simulink model "test_7x7x7_timing"  (R2013b)
settings: Solver=ode3  SolverMode=SingleTasking  StartTime=0.0  StopTime=inf  RelTol=1e-3
InitFcn:
  | close all
model workspace (MAT data in the model file):
  dt = 0.003
libraries: arduinolib x97, simulink x8, rtwinlib x1
settings Model: ExtModeTrigDuration=2  Creator=sbiagion  LastModifiedBy=sbiagion
settings DataIOCC: SignalLoggingSaveFormat=ModelDataLogs
settings OptimizationCC: OptimizeModelRefInitCode=on  LifeSpan=1
settings DebuggingCC: SolverPrmCheckMsg=none  MultiTaskDSMMsg=warning  MultiTaskCondExecSysMsg=none
settings HardwareCC: ProdBitPerInt=16  ProdBitPerPointer=8  ProdIntDivRoundTo=Zero  ProdEndianess=LittleEndian  ProdWordSize=8  ProdHWDeviceType=Atmel->AVR
settings RTWCC: SystemTargetFile=realtime.tlc  GenerateMakefile=off  TemplateMakefile=realtime.tmf  Description=Run on Target Hardware  RTWVerbose=off  ProcessScript=realtime_make_rtw_hook  IncludeERTFirstTime=on
settings STFCustomTargetCC: TargetLibSuffix=.a  GenerateSampleERTMain=on  ERTCustomFileBanners=on  SupportNonInlinedSFcns=off  SupportVariableSizeSignals=on  MATLABClassNameForMDSCustomization=Simulink.SoftwareTarget.ERTCustomization  GRTInterface=off  SystemTargetFile=realtime.tlc
settings ERTTargetCC: CodeReplacementLibrary=ANSI_C  GenerateSampleERTMain=on  ParMdlRefBuildCompliant=off  CompOptLevelCompliant=off  ConcurrentExecutionCompliant=off  CombineOutputUpdateFcns=off  ERTFirstTimeCompliant=off  SupportContinuousTime=on  SupportVariableSizeSignals=on  ModelStepFunctionPrototypeControlCompliant=off  CPPClassGenCompliant=off  ExtMode=on  ExtModeTransport=3  ExtModeMexFile=ext_serial_win32_comm  ExtModeMexArgs=0 18 115200  InlinedParameterPlacement=NonHierarchical  ERTSrcFileBannerTemplate=realtime_code_template.cgt  ERTHdrFileBannerTemplate=realtime_code_template.cgt  ERTDataSrcFileTemplate=realtime_code_template.cgt  ERTDataHdrFileTemplate=realtime_code_template.cgt  ERTCustomFileTemplate=realtime_file_process.tlc

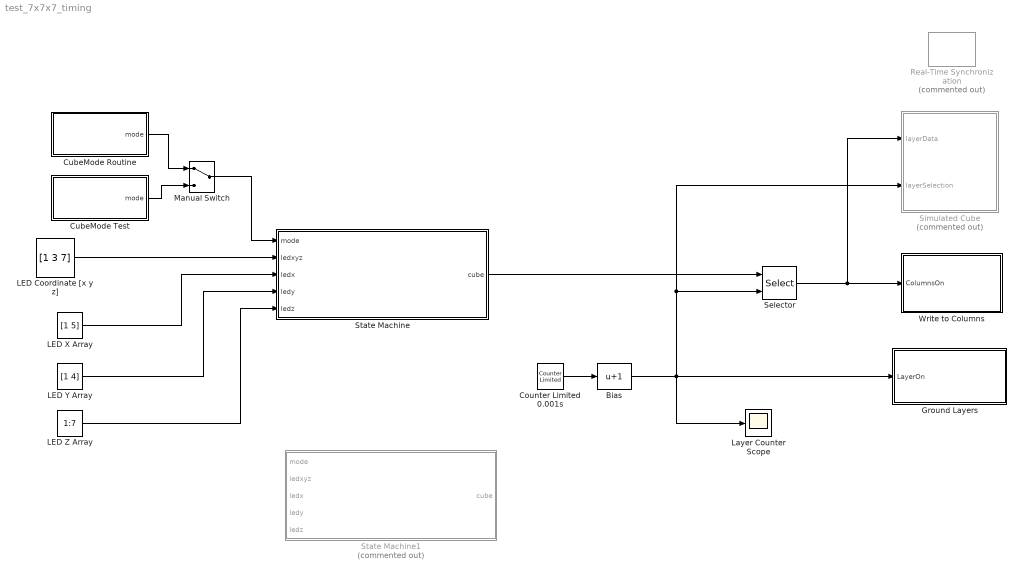
== system test_7x7x7_timing ==
  Bias : Bias  Bias=1
  Counter Limited 0.001s : simulink/Sources/Counter Limited  uplimit=6  tsamp=dt
  CubeMode Routine : Stateflow chart  TreatAsAtomicUnit=on
  CubeMode Test : Stateflow chart  TreatAsAtomicUnit=on
  Ground Layers : Subsystem
  LED Coordinate [x y z] : Constant  Value=[1 3 7]  SampleTime=-1
  LED X Array : Constant  Value=[1 5]
  LED Y Array : Constant  Value=[1 4]
  LED Z Array : Constant  Value=1:7
  Layer Counter Scope : Scope
      settings: TimeRange=20  YMin=-1  YMax=7
  Manual Switch : ManualSwitch
  Real-Time Synchronization : rtwinlib/Real-Time Synchronization  Commented=on  SampleTime=1  MaxMissedTicks=1000  ShowMissedTicks=off  YieldWhenWaiting=on
  Selector : Selector  NumberOfDimensions=3  InputPortWidth=3  SampleTime=dt  IndexOptions=Select all,Select all,Index vector (port)  Indices=1:7,1:7,1  OutputSizes=1,1,1
  Simulated Cube : MATLAB Function  Commented=on  TreatAsAtomicUnit=on
  State Machine : Stateflow chart  TreatAsAtomicUnit=on  SystemSampleTime=0.1
  State Machine1 : Stateflow chart  Commented=on  TreatAsAtomicUnit=on  SystemSampleTime=0.1
  Write to Columns : Subsystem
  wires:
  CubeMode Test/1(mode) -> Manual Switch/2
  State Machine/1(cube) -> Selector/1
  Counter Limited 0.001s/1 -> Bias/1
  LED Coordinate [x y z]/1 -> State Machine/2(ledxyz)
  Selector/1 -> Simulated Cube/1(layerData), Write to Columns/1(ColumnsOn)
  LED X Array/1 -> State Machine/3(ledx)
  LED Y Array/1 -> State Machine/4(ledy)
  LED Z Array/1 -> State Machine/5(ledz)
  Bias/1 -> Simulated Cube/2(layerSelection), Selector/2, Ground Layers/1(LayerOn), Layer Counter Scope/1
  CubeMode Routine/1(mode) -> Manual Switch/1
  Manual Switch/1 -> State Machine/1(mode)

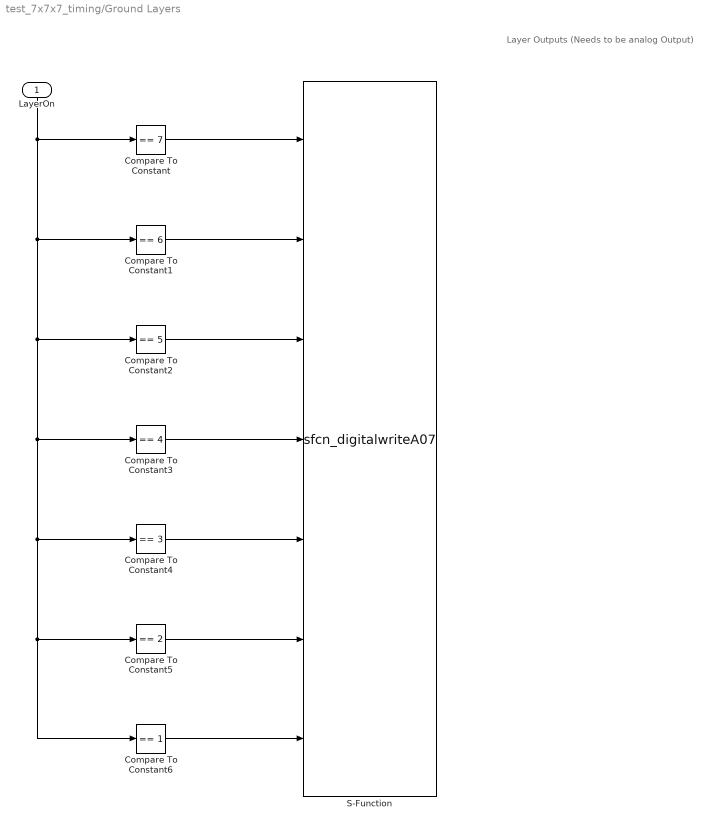
== system test_7x7x7_timing/Ground Layers ==
  note: Layer Outputs (Needs to be analog Output)
  LayerOn : Inport
  Compare To Constant : simulink/Logic and Bit Operations/Compare To Constant  relop===  const=7  OutDataTypeStr=uint8
  Compare To Constant1 : simulink/Logic and Bit Operations/Compare To Constant  relop===  const=6  OutDataTypeStr=uint8
  Compare To Constant2 : simulink/Logic and Bit Operations/Compare To Constant  relop===  const=5  OutDataTypeStr=uint8
  Compare To Constant3 : simulink/Logic and Bit Operations/Compare To Constant  relop===  const=4  OutDataTypeStr=uint8
  Compare To Constant4 : simulink/Logic and Bit Operations/Compare To Constant  relop===  const=3  OutDataTypeStr=uint8
  Compare To Constant5 : simulink/Logic and Bit Operations/Compare To Constant  relop===  const=2  OutDataTypeStr=uint8
  Compare To Constant6 : simulink/Logic and Bit Operations/Compare To Constant  relop===  const=1  OutDataTypeStr=uint8
  S-Function : S-Function  FunctionName=sfcn_digitalwriteA07  Parameters=0  EnableBusSupport=off
  wires:
  LayerOn/1 -> Compare To Constant6/1, Compare To Constant5/1, Compare To Constant4/1, Compare To Constant3/1, Compare To Constant2/1, Compare To Constant1/1, Compare To Constant/1
  Compare To Constant/1 -> S-Function/1
  Compare To Constant1/1 -> S-Function/2
  Compare To Constant2/1 -> S-Function/3
  Compare To Constant3/1 -> S-Function/4
  Compare To Constant4/1 -> S-Function/5
  Compare To Constant5/1 -> S-Function/6
  Compare To Constant6/1 -> S-Function/7

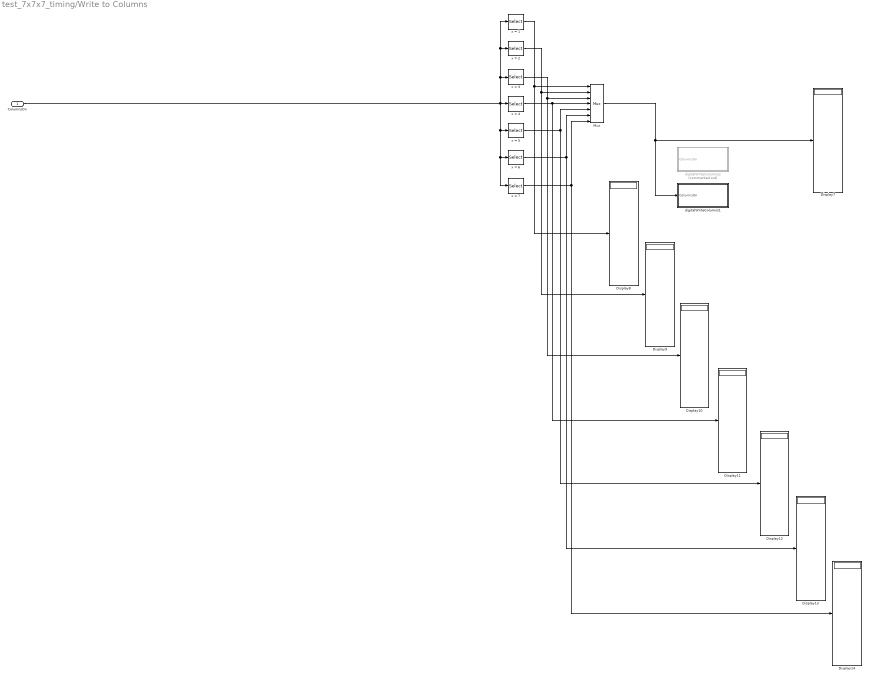
== system test_7x7x7_timing/Write to Columns ==
  ColumnsOn : Inport
  Display{7..14} (8 alike) : Display
  Mux : Mux  Inputs=7
  digitalWriteColumns1 : Subsystem
  digitalWriteColumns2 : Subsystem  Commented=on
  x = 1 : Selector  NumberOfDimensions=2  InputPortWidth=49  IndexOptions=Index vector (dialog),Select all  Indices=1,1  OutputSizes=1,1
  x = 2 : Selector  NumberOfDimensions=2  InputPortWidth=49  IndexOptions=Index vector (dialog),Select all  Indices=2,2  OutputSizes=1,1
  x = 3 : Selector  NumberOfDimensions=2  InputPortWidth=49  IndexOptions=Index vector (dialog),Select all  Indices=3,3  OutputSizes=1,1
  x = 4 : Selector  NumberOfDimensions=2  InputPortWidth=49  IndexOptions=Index vector (dialog),Select all  Indices=4,4  OutputSizes=1,1
  x = 5 : Selector  NumberOfDimensions=2  InputPortWidth=49  IndexOptions=Index vector (dialog),Select all  Indices=5,5  OutputSizes=1,1
  x = 6 : Selector  NumberOfDimensions=2  InputPortWidth=49  IndexOptions=Index vector (dialog),Select all  Indices=6,6  OutputSizes=1,1
  x = 7 : Selector  NumberOfDimensions=2  InputPortWidth=49  IndexOptions=Index vector (dialog),Select all  Indices=7,7  OutputSizes=1,1
  wires:
  x = 1/1 -> Display8/1, Mux/1
  x = 2/1 -> Display9/1, Mux/2
  x = 3/1 -> Mux/3, Display10/1
  ColumnsOn/1 -> x = 1/1, x = 2/1, x = 3/1, x = 4/1, x = 5/1, x = 7/1, x = 6/1
  x = 6/1 -> Mux/6, Display13/1
  x = 5/1 -> Mux/5, Display12/1
  Mux/1 -> digitalWriteColumns1/1(ColumnsOn), Display7/1
  x = 7/1 -> Mux/7, Display14/1
  x = 4/1 -> Mux/4, Display11/1

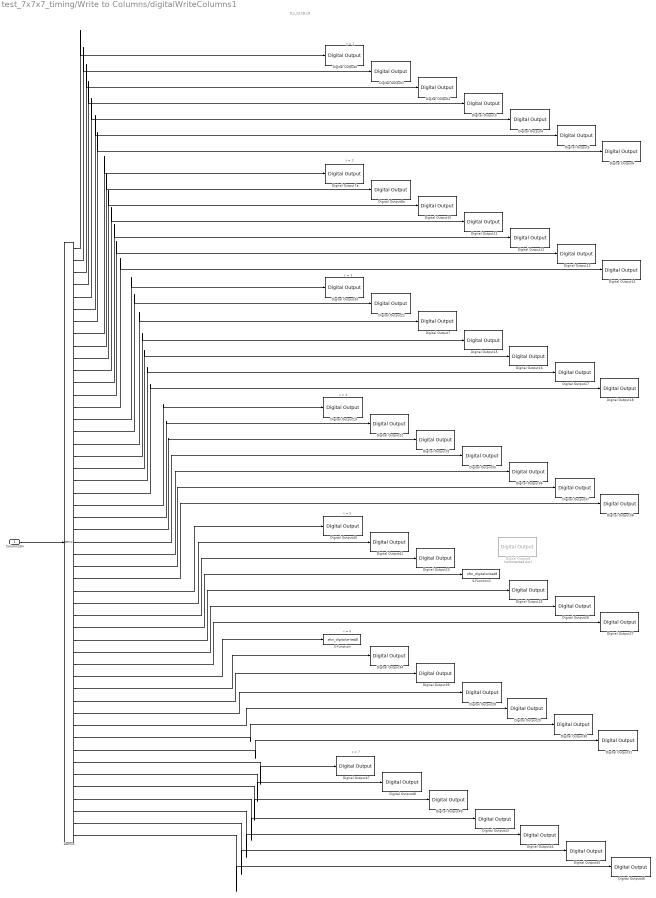
== system test_7x7x7_timing/Write to Columns/digitalWriteColumns1 ==
  note: 0,1,13,18,19
  note: x = 7
  note: x = 6
  note: x = 5
  note: x = 4
  note: x = 3
  note: x = 2
  note: x = 1
  ColumnsOn : Inport
  Demux : Demux  Outputs=49
  Digital Output0 : arduinolib/Digital Output  pinNumber=38
  Digital Output1 : arduinolib/Digital Output  pinNumber=40
  Digital Output10 : arduinolib/Digital Output  pinNumber=44
  Digital Output11 : arduinolib/Digital Output  pinNumber=35
  Digital Output12 : arduinolib/Digital Output  pinNumber=45
  Digital Output13 : arduinolib/Digital Output  pinNumber=32
  Digital Output14 : arduinolib/Digital Output  pinNumber=46
  Digital Output15 : arduinolib/Digital Output  pinNumber=48
  Digital Output16 : arduinolib/Digital Output  pinNumber=31
  Digital Output17 : arduinolib/Digital Output  pinNumber=49
  Digital Output18 : arduinolib/Digital Output  pinNumber=28
  Digital Output19 : arduinolib/Digital Output  pinNumber=50
  Digital Output2 : arduinolib/Digital Output  pinNumber=39
  Digital Output20 : arduinolib/Digital Output  pinNumber=33
  Digital Output21 : arduinolib/Digital Output  pinNumber=47
  Digital Output22 : arduinolib/Digital Output  pinNumber=29
  Digital Output23 : arduinolib/Digital Output  pinNumber=22
  Digital Output25 : arduinolib/Digital Output  pinNumber=25
  Digital Output26 : arduinolib/Digital Output  pinNumber=8
  Digital Output27 : arduinolib/Digital Output  pinNumber=24
  Digital Output28 : arduinolib/Digital Output  pinNumber=10
  Digital Output29 : arduinolib/Digital Output  pinNumber=4
  Digital Output3 : arduinolib/Digital Output  pinNumber=41
  Digital Output30 : arduinolib/Digital Output  pinNumber=9
  Digital Output31 : arduinolib/Digital Output  pinNumber=5
  Digital Output32 : arduinolib/Digital Output  pinNumber=51
  Digital Output34 : arduinolib/Digital Output  pinNumber=21
  Digital Output35 : arduinolib/Digital Output  pinNumber=26
  Digital Output36 : arduinolib/Digital Output  pinNumber=52
  Digital Output37 : arduinolib/Digital Output  pinNumber=27
  Digital Output38 : arduinolib/Digital Output  pinNumber=53
  Digital Output39 : arduinolib/Digital Output  pinNumber=3
  Digital Output4 : arduinolib/Digital Output  pinNumber=36
  Digital Output40 : arduinolib/Digital Output  pinNumber=23
  Digital Output41 : arduinolib/Digital Output  pinNumber=6
  Digital Output43 : arduinolib/Digital Output  pinNumber=11
  Digital Output44 : arduinolib/Digital Output  pinNumber=17
  Digital Output45 : arduinolib/Digital Output  pinNumber=12
  Digital Output46 : arduinolib/Digital Output  pinNumber=20
  Digital Output47 : arduinolib/Digital Output  pinNumber=15
  Digital Output48 : arduinolib/Digital Output  pinNumber=14
  Digital Output49 : arduinolib/Digital Output  pinNumber=16
  Digital Output5 : arduinolib/Digital Output  pinNumber=42
  Digital Output6 : arduinolib/Digital Output  pinNumber=37
  Digital Output7 : arduinolib/Digital Output  pinNumber=30
  Digital Output7a : arduinolib/Digital Output  pinNumber=43
  Digital Output8 : arduinolib/Digital Output  Commented=on  pinNumber=7
  Digital Output8a : arduinolib/Digital Output  pinNumber=34
  S-Function : S-Function  FunctionName=sfcn_digitalwriteA8  Parameters=0  EnableBusSupport=off
  S-Function1 : S-Function  FunctionName=sfcn_digitalwriteA9  Parameters=0  EnableBusSupport=off
  wires:
  Demux/4 -> Digital Output3/1
  ColumnsOn/1 -> Demux/1
  Demux/3 -> Digital Output2/1
  Demux/2 -> Digital Output1/1
  Demux/1 -> Digital Output0/1
  Demux/7 -> Digital Output6/1
  Demux/6 -> Digital Output5/1
  Demux/5 -> Digital Output4/1
  Demux/11 -> Digital Output11/1
  Demux/10 -> Digital Output10/1
  Demux/9 -> Digital Output8a/1
  Demux/8 -> Digital Output7a/1
  Demux/14 -> Digital Output14/1
  Demux/13 -> Digital Output13/1
  Demux/12 -> Digital Output12/1
  Demux/18 -> Digital Output15/1
  Demux/17 -> Digital Output7/1
  Demux/16 -> Digital Output21/1
  Demux/15 -> Digital Output20/1
  Demux/21 -> Digital Output18/1
  Demux/20 -> Digital Output17/1
  Demux/19 -> Digital Output16/1
  Demux/25 -> Digital Output35/1
  Demux/24 -> Digital Output32/1
  Demux/23 -> Digital Output22/1
  Demux/22 -> Digital Output19/1
  Demux/28 -> Digital Output38/1
  Demux/27 -> Digital Output37/1
  Demux/26 -> Digital Output36/1
  Demux/32 -> S-Function1/1
  Demux/31 -> Digital Output23/1
  Demux/30 -> Digital Output41/1
  Demux/29 -> Digital Output40/1
  Demux/35 -> Digital Output27/1
  Demux/34 -> Digital Output26/1
  Demux/33 -> Digital Output25/1
  Demux/39 -> Digital Output28/1
  Demux/38 -> Digital Output39/1
  Demux/37 -> Digital Output34/1
  Demux/36 -> S-Function/1
  Demux/42 -> Digital Output31/1
  Demux/41 -> Digital Output30/1
  Demux/40 -> Digital Output29/1
  Demux/46 -> Digital Output43/1
  Demux/45 -> Digital Output49/1
  Demux/44 -> Digital Output48/1
  Demux/43 -> Digital Output47/1
  Demux/49 -> Digital Output46/1
  Demux/48 -> Digital Output45/1
  Demux/47 -> Digital Output44/1

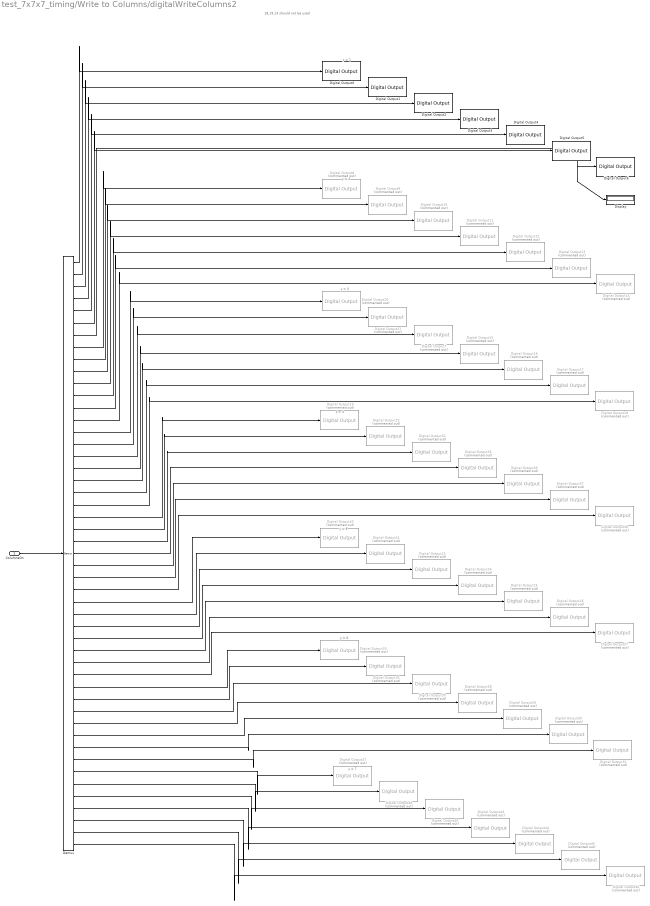
== system test_7x7x7_timing/Write to Columns/digitalWriteColumns2 ==
  note: y = 1
  note: y = 2
  note: y = 3
  note: y = 4
  note: y = 5
  note: y = 6
  note: y = 7
  note: 18,19,13 should not be used
  ColumnsOn : Inport
  Demux : Demux  Outputs=49
  Digital Output0 : arduinolib/Digital Output  pinNumber=2
  Digital Output1 : arduinolib/Digital Output  pinNumber=3
  Digital Output10 : arduinolib/Digital Output  Commented=on  pinNumber=9
  Digital Output11 : arduinolib/Digital Output  Commented=on  pinNumber=10
  Digital Output12 : arduinolib/Digital Output  Commented=on  pinNumber=11
  Digital Output13 : arduinolib/Digital Output  Commented=on  pinNumber=49
  Digital Output14 : arduinolib/Digital Output  Commented=on  pinNumber=50
  Digital Output15 : arduinolib/Digital Output  Commented=on  pinNumber=15
  Digital Output16 : arduinolib/Digital Output  Commented=on  pinNumber=16
  Digital Output17 : arduinolib/Digital Output  Commented=on  pinNumber=17
  Digital Output18 : arduinolib/Digital Output  Commented=on  pinNumber=18
  Digital Output19 : arduinolib/Digital Output  Commented=on  pinNumber=19
  Digital Output2 : arduinolib/Digital Output  pinNumber=4
  Digital Output20 : arduinolib/Digital Output  Commented=on  pinNumber=12
  Digital Output21 : arduinolib/Digital Output  Commented=on  pinNumber=51
  Digital Output22 : arduinolib/Digital Output  Commented=on  pinNumber=20
  Digital Output23 : arduinolib/Digital Output  Commented=on  pinNumber=28
  Digital Output24 : arduinolib/Digital Output  Commented=on  pinNumber=29
  Digital Output25 : arduinolib/Digital Output  Commented=on  pinNumber=30
  Digital Output26 : arduinolib/Digital Output  Commented=on  pinNumber=31
  Digital Output27 : arduinolib/Digital Output  Commented=on  pinNumber=32
  Digital Output28 : arduinolib/Digital Output  Commented=on  pinNumber=36
  Digital Output29 : arduinolib/Digital Output  Commented=on  pinNumber=37
  Digital Output3 : arduinolib/Digital Output  pinNumber=5
  Digital Output30 : arduinolib/Digital Output  Commented=on  pinNumber=38
  Digital Output31 : arduinolib/Digital Output  Commented=on  pinNumber=39
  Digital Output32 : arduinolib/Digital Output  Commented=on  pinNumber=21
  Digital Output33 : arduinolib/Digital Output  Commented=on  pinNumber=33
  Digital Output34 : arduinolib/Digital Output  Commented=on  pinNumber=34
  Digital Output35 : arduinolib/Digital Output  Commented=on  pinNumber=22
  Digital Output36 : arduinolib/Digital Output  Commented=on  pinNumber=23
  Digital Output37 : arduinolib/Digital Output  Commented=on  pinNumber=24
  Digital Output38 : arduinolib/Digital Output  Commented=on  pinNumber=25
  Digital Output39 : arduinolib/Digital Output  Commented=on  pinNumber=35
  Digital Output4 : arduinolib/Digital Output  pinNumber=6
  Digital Output40 : arduinolib/Digital Output  Commented=on  pinNumber=26
  Digital Output41 : arduinolib/Digital Output  Commented=on  pinNumber=27
  Digital Output43 : arduinolib/Digital Output  Commented=on  pinNumber=43
  Digital Output44 : arduinolib/Digital Output  Commented=on  pinNumber=44
  Digital Output45 : arduinolib/Digital Output  Commented=on  pinNumber=45
  Digital Output46 : arduinolib/Digital Output  Commented=on  pinNumber=46
  Digital Output47 : arduinolib/Digital Output  Commented=on  pinNumber=40
  Digital Output48 : arduinolib/Digital Output  Commented=on  pinNumber=41
  Digital Output49 : arduinolib/Digital Output  Commented=on  pinNumber=42
  Digital Output5 : arduinolib/Digital Output  pinNumber=7
  Digital Output6 : arduinolib/Digital Output  pinNumber=53
  Digital Output7 : arduinolib/Digital Output  Commented=on  pinNumber=14
  Digital Output8 : arduinolib/Digital Output  Commented=on  pinNumber=7
  Digital Output9 : arduinolib/Digital Output  Commented=on  pinNumber=8
  Display : Display
  wires:
  Demux/47 -> Digital Output44/1
  Demux/48 -> Digital Output45/1
  Demux/49 -> Digital Output46/1
  Demux/43 -> Digital Output47/1
  Demux/44 -> Digital Output48/1
  Demux/45 -> Digital Output49/1
  Demux/46 -> Digital Output43/1
  Demux/40 -> Digital Output29/1
  Demux/41 -> Digital Output30/1
  Demux/42 -> Digital Output31/1
  Demux/36 -> Digital Output33/1
  Demux/37 -> Digital Output34/1
  Demux/38 -> Digital Output39/1
  Demux/39 -> Digital Output28/1
  Demux/33 -> Digital Output25/1
  Demux/34 -> Digital Output26/1
  Demux/35 -> Digital Output27/1
  Demux/29 -> Digital Output40/1
  Demux/30 -> Digital Output41/1
  Demux/31 -> Digital Output23/1
  Demux/32 -> Digital Output24/1
  Demux/26 -> Digital Output36/1
  Demux/27 -> Digital Output37/1
  Demux/28 -> Digital Output38/1
  Demux/22 -> Digital Output19/1
  Demux/23 -> Digital Output22/1
  Demux/24 -> Digital Output32/1
  Demux/25 -> Digital Output35/1
  Demux/19 -> Digital Output16/1
  Demux/20 -> Digital Output17/1
  Demux/21 -> Digital Output18/1
  Demux/15 -> Digital Output20/1
  Demux/16 -> Digital Output21/1
  Demux/17 -> Digital Output7/1
  Demux/18 -> Digital Output15/1
  Demux/12 -> Digital Output12/1
  Demux/13 -> Digital Output13/1
  Demux/14 -> Digital Output14/1
  Demux/8 -> Digital Output8/1
  Demux/9 -> Digital Output9/1
  Demux/10 -> Digital Output10/1
  Demux/11 -> Digital Output11/1
  Demux/5 -> Digital Output4/1
  Demux/6 -> Digital Output5/1
  Demux/7 -> Digital Output6/1, Display/1
  Demux/1 -> Digital Output0/1
  Demux/2 -> Digital Output1/1
  Demux/3 -> Digital Output2/1
  ColumnsOn/1 -> Demux/1
  Demux/4 -> Digital Output3/1

== stateflow chart test_7x7x7_timing/CubeMode Routine ==
  state InitializeOff
    entry:
    mode = 1;
  state StarMode
    % 0:30 End of Basic Stage and Start of Yoshi Ride
    entry:
    mode = 7;
  state HeartMode
    % 1:05 Start of Double Seesaw
    entry:
    mode = 8;
  state TurnOff
    % end at 2:05
    entry: mode = 1;
  state FireworksMode
    % 1:45 End of Seesaw, starting at 1:35
    entry:
    mode = 9;
  (default) -> InitializeOff : % turn on 30s before NXT moves
  InitializeOff -> StarMode : after(60,sec)
  StarMode -> HeartMode : after(35,sec)
  FireworksMode -> TurnOff : after(30,sec)
  HeartMode -> FireworksMode : after(30,sec)
  data: mode output

== matlab function test_7x7x7_timing/Simulated Cube ==
  data: layerData input; layerSelection input
function simulatedCube(layerData,layerSelection)

coder.extrinsic('set','drawnow');

persistent cube t;

if isempty(cube)
  nLEDpDim = 7;
  
  t = 0;
  cube.nLEDpDim = nLEDpDim;
  fh = figure;
  set(fh,'renderer','opengl'); % if you close the figure window while the
                               % simulation is running, MATLAB will crash.
  ah = axes;
  xlabel('x-axis');
  ylabel('y-axis');
  zlabel('z-axis');
  set(ah,...
    'xLim',[0 nLEDpDim+1],...
    'yLim',[0 nLEDpDim+1],...
    'zLim',[0 nLEDpDim+1]);
  view(3);
  axis vis3d;
  grid on;
  set(ah,'XTick',[0 1 2 3 4 5 6 7 8])
  set(ah,'YTick',[0 1 2 3 4 5 6 7 8])
  set(ah,'ZTick',[0 1 2 3 4 5 6 7 8])
  cube.LED = zeros(nLEDpDim,nLEDpDim,nLEDpDim);
  for i = 1:nLEDpDim^3
    cube.LED(i) = line(0,0,0,...
      'parent',ah,...
      'color',[0.8,0.1,0.1],...
      'visible','off',...
      'marker','.',...
      'markerSize',15);
  end
  for i = 1:nLEDpDim
    set(cube.LED(i,:,:),'xData',i);
    set(cube.LED(:,i,:),'yData',i);
    set(cube.LED(:,:,i),'zData',i);
  end
end

if ~mod(t,1)
  set(cube.LED(:,:,mod(int8(layerSelection)-1,cube.nLEDpDim)+1),...
    'visible','off');
  activeLayer = cube.LED(:,:,layerSelection);
  activeLED   = activeLayer(logical(layerData));
  set(activeLED,'visible','on');
  drawnow;
end
t = t + 1;

== stateflow chart test_7x7x7_timing/State Machine ==
  state AllOff
    % All LED's off
    entry: cube = false(7,7,7);
  state Star
    %Star
    state MoveAlongPlane
      state Normal2Y
        state MoveAlongY
          en:
          j = j+1;
          if j==8
          j = 1;
          end
        state DrawStarY
          entry:
          % draw star normal to Y-axis
          cube  = drawStar(2,j);
        (default) -> DrawStarY : {j = 1;}
        DrawStarY -> MoveAlongY : after(0.1,sec)
        MoveAlongY -> DrawStarY
      state Normal2X
        state MoveAlongX
          en:
          i = i+1;
          if i==8
          i = 1;
          end
        state DrawStarX
          entry:
          cube  = drawStar(1,i);
        (default) -> DrawStarX : {i = 1;}
        DrawStarX -> MoveAlongX : after(0.1,sec)
        MoveAlongX -> DrawStarX
      (default) -> Star.MoveAlongPlane.Normal2Y
      Star.MoveAlongPlane.Normal2Y -> Star.MoveAlongPlane.Normal2X : after(5,sec)
      Star.MoveAlongPlane.Normal2X -> Star.MoveAlongPlane.Normal2Y : after(5,sec)
    state RotateSprite
      state normalToY
        entry:
        cube = rotateSprite(cube,'z','y',rStep);
      state Wait1
      state normalToX
        entry:
        cube = rotateSprite(cube,'z','x',rStep);
      state Wait2
      (default) -> Wait1 : {% draw star normal to y-axis
          | cube  = drawStar(1,4);
          | rStep = 1;}
      Wait1 -> normalToY [order 1] : [after(0.7,sec)]
      normalToY -> Wait1 : {rStep = rStep + 1;}
      Wait1 -> (junction 429) [order 2] : [rStep == 9]
      (junction 430) -> Wait1 : {rStep = 1;}
      (junction 429) -> Wait2 : {rStep = 1;}
      Wait2 -> (junction 430) [order 1] : [rStep == 9]
      Wait2 -> normalToX [order 2] : [after(0.7,sec)]
      normalToX -> Wait2 : {rStep = rStep + 1}
    (default) -> MoveAlongPlane
    MoveAlongPlane -> RotateSprite : after(20,sec)
  state Heart
    %Star
    state Normal2Y
      state drawNormal2Y
        entry: cube = drawHeart(2,4);
      state heartBeat
        entry: cube = drawHeartBeat(2,4);
      (default) -> drawNormal2Y
      drawNormal2Y -> Heart.Normal2Y.heartBeat : after(1.5,sec)
      Heart.Normal2Y.heartBeat -> drawNormal2Y : after(0.5,sec)
    state Normal2X
      state drawNormal2X
        entry: cube = drawHeart(1,4);
      state heartBeat
        entry: cube = drawHeartBeat(1,4);
      (default) -> drawNormal2X
      drawNormal2X -> Heart.Normal2X.heartBeat : after(1.5,sec)
      Heart.Normal2X.heartBeat -> drawNormal2X : after(0.5,sec)
    (default) -> Heart.Normal2Y
    Heart.Normal2Y -> Heart.Normal2X : after(10,sec)
    Heart.Normal2X -> Heart.Normal2Y : after(10,sec)
  state Firecrackers
    state LongWait
    state EvolveAnimation
      entry:
      cube = fireworks(cube,rStep,exp);
      exit:
      rStep = mod(rStep,21)+1;
    state ShortWait
      % Explosion
    (default) -> LongWait : {cube  = false(7,7,7);
        | exp = drawExplosion;
        | rStep = 1;}
    EvolveAnimation -> ShortWait [order 2] : [rStep > 8 && rStep < 15]
    LongWait -> EvolveAnimation : [after(0.1,sec)]
    ShortWait -> EvolveAnimation : [after(0.10,sec)]
    EvolveAnimation -> LongWait [order 1] : [rStep < 9 || rStep >14]
  state debug
  (default) -> (junction 73) : {cube = false(7,7,7);}
  (junction 69) -> (junction 73)
  (junction 73) -> (junction 402)
  (junction 400) -> (junction 69)
  (junction 402) -> AllOff [order 1] : [mode==1]
  (junction 402) -> (junction 455) [order 2]
  AllOff -> (junction 400) : [mode~=1]
  (junction 404) -> (junction 400)
  (junction 455) -> Star [order 1] : [mode==7]
  Star -> (junction 404) : [mode~=7]
  (junction 455) -> (junction 586) [order 2]
  (junction 585) -> (junction 404)
  (junction 586) -> Heart [order 1] : [mode==8]
  Heart -> (junction 585) : [mode~=8]
  (junction 586) -> (junction 470) [order 2]
  (junction 464) -> (junction 585)
  (junction 470) -> Firecrackers [order 1] : [mode==9]
  Firecrackers -> (junction 464) : [mode~=9]
  (junction 470) -> debug [order 2]
  data: cubeout function_output; axis function_input; coord function_input; bin function_input; rotationAxis function_input; normalAxis function_input; step function_input; b function_output; cubeout function_output; axis function_input; coord function_input; cubeout function_output; axis function_input; coord function_input; explosion function_output; cubeIn function_input; step function_input; cubeOut function_output; explosion function_input; mode input; ledxyz input; cube output size=[7 7 7]; yi local; xi local; ledx input; ledy input; ledz input; rStep local; j local; i local; exp local
  function cubeout = drawStar(axis,coord):
    | function cubeout = drawStar(axis,coord)
    |     cubeout = false(7,7,7);
    |     cubeyi = [0 0 0 1 0 0 0
    |               0 0 1 1 1 0 0;
    |               1 1 1 1 1 1 1;
    |               0 0 1 1 1 0 0;
    |               0 1 1 1 1 1 0;
    |               0 1 1 0 1 1 0;
    |               1 0 0 0 0 0 1];
    |      cubeyi = rot90(cubeyi,3);
    |     % draw normal to x axis, i.e. in y-z plane
    |     if axis == 1 
    |         for ii = coord(1):coord(end)
    |                 cubeout(ii,:,:) = cubeyi;
    |         end
    |     % draw normal to y-axis, i.e. in x-z plane
    |     elseif axis == 2
    |             for ii = coord(1):coord(end)
    |                 cubeout(:,ii,:) = cubeyi;
    |             end
    |     % draw normal to z-axis, i.e. in x-y plane
    |     elseif axis == 3;
    |             for ii = coord(1):coord(end)
    |                 cubeout(:,:,ii) = cubeyi;
    |             end
    |     end
  function b = rotateSprite(bin,rotationAxis,normalAxis,step):
    | function b = rotateSprite(bin,rotationAxis,normalAxis,step)
    | % Rotate a sprite laying in the plane normal to 'normalAxis' about
    | % 'rotationAxis' by a quarter turn. This function must be called 8 times
    | % with increasing values of 'step' from 1 to 8 to complete the quarter
    | % turn. The sprite must lie in a central plane of the LED cube.
    | %
    | % Frame of reference.
    | % The origin is at b(1,1,1), an LED on the top corner of the cube.
    | % X axis increases from b(1,1,1) to b(1,7,1)
    | % Y axis increases from b(1,1,1) to b(7,1,1)
    | % Z axis increases from b(1,1,1) to b(1,1,7), an LED on the bottom corner
    | %
    | % Inputs and outputs.
    | % b : LED matrix
    | % rotationAxis : 'x', 'y', or 'z'
    | % normalAxis : 'x', 'y', or 'z'
    | % step : integer in the set 1:8
    | %
    | % Example.
    | % b = zeros(7,7,7);
    | % b(4,:,:) = 1;
    | % b = rotateSprite(b,'z','y',1)
    | % b = rotateSprite(b,'z','y',2)
    | % ...
    | % b = rotateSprite(b,'z','y',8)
    | 
    | % Transform b so that all rotations are equivalent to the case where the
    | % sprite is normal to the 'y' axis and the rotation is about the 'z' axis.
    | % After the rotation is performed, transform the LED back.
    | if     strcmp(rotationAxis,'z') && strcmp(normalAxis,'y')
    |   p = [1 2 3];
    |   mirrorDim = 2;
    | elseif strcmp(rotationAxis,'z') && strcmp(normalAxis,'x')
    |   p = [2 1 3];
    |   mirrorDim = 3;
    | elseif strcmp(rotationAxis,'y') && strcmp(normalAxis,'x')
    |   p = [2 3 1];
    |   mirrorDim = 2;
    | elseif strcmp(rotationAxis,'y') && strcmp(normalAxis,'z')
    |   p = [3 2 1];
    |   mirrorDim = 1;
    | elseif strcmp(rotationAxis,'x') && strcmp(normalAxis,'z')
    |   p = [3 1 2];
    |   mirrorDim = 1;
    | else % strcmp(rotationAxis,'x') && strcmp(normalAxis,'y')
    |   p = [1 3 2];
    |   mirrorDim = 2;  
    | end
    | 
    | b = permute(bin,p);
    | b = flipdim(b,mirrorDim);
    | 
    | % Assume sprite is normal to (0 1 0) y axis and to be rotated about
    | % the (0 0 1) z axis.
    | if     (step == 1) 
    |   b = pushPixels(b,...
    |     [4 1; 4 7],... % LEDs' values to push.
    |     [5 1; 3 7]);   % LEDs to recieve pushed values.
    | elseif (step == 2)
    |   b = pushPixels(b,...
    |     [4 2; 4 6],...
    |     [5 2; 3 6]);
    | elseif (step == 3)
    |   b = pushPixels(b,...
    |     [5 1; 3 7; 4 3; 4 5],...
    |     [6 1; 2 7; 5 3; 3 5]);
    | elseif (step == 4) % after this, sprite is normal to (1 1 0)
    |   b = pushPixels(b,...
    |     [6 1; 5 2; 2 7; 3 6],...
    |     [7 1; 6 2; 1 7; 2 6]);
    | elseif (step == 5) % now reverse the steps above and swap x with y
    |   b = pushPixels(b,...
    |     fliplr([7 1; 6 2; 1 7; 2 6]),...
    |     fliplr([6 1; 5 2; 2 7; 3 6]));
    | elseif (step == 6)
    |   b = pushPixels(b,...
    |     fliplr([6 1; 2 7; 5 3; 3 5]),...
    |     fliplr([5 1; 3 7; 4 3; 4 5]));
    | elseif (step == 7)
    |   b = pushPixels(b,...
    |     fliplr([5 2; 3 6]),...
    |     fliplr([4 2; 4 6]));
    | else% (step == 8) % after this, sprite will be orthogonal to initial position
    |   b = pushPixels(b,...
    |     fliplr([5 1; 3 7]),...
    |     fliplr([4 1; 4 7]));
    | end
    | 
    | % Inverse transformations to restore the frame of reference
    | b = ipermute(b,p);
    | b = flipdim(b,mirrorDim);
    | 
    | end
    | 
    | 
    | function b = pushPixels(b,prevLED,nextLED)
    | % Push the values of LED(prevInd) to LED(nextInd), then shut off
    | % LED(prevInd). Perform this transformation for all layers of b. The
    | % transformation is the same for all layers.
    | %
    | % b       : matrix of LEDs
    | % prevLED : n by 2 matrix of [row,col] indices.
    | % nextLED : same as prevLED.
    | 
    | matrixSize = size(b);
    | numLayers = size(b,3);
    | allLayers = reshape(repmat(1:numLayers,size(nextLED,1),1),[],1);
    | 
    |   next = sub2ind(matrixSize,...
    |     repmat(nextLED(:,1),numLayers,1),...
    |     repmat(nextLED(:,2),numLayers,1),...
    |     allLayers); % next LEDs to turn on.
    |   prev = sub2ind(matrixSize,...
    |     repmat(prevLED(:,1),numLayers,1),...
    |     repmat(prevLED(:,2),numLayers,1),...
    |     allLayers); % previous LEDs to turn off.
    |   b(next) = b(prev);
    |   b(prev) = 0;
    | end
  function cubeout = drawHeart(axis,coord):
    | function cubeout = drawHeart(axis,coord)
    |     cubeout = false(7,7,7);
    |     cubei = [0 0 0 0 0 0 0
    |               0 1 1 0 1 1 0;
    |               1 1 1 1 1 1 1;
    |               1 1 1 1 1 1 1;
    |               0 1 1 1 1 1 0;
    |               0 0 1 1 1 0 0;
    |               0 0 0 1 0 0 0];
    |      cubei = rot90(cubei,3);
    |     % draw normal to x axis, i.e. in y-z plane
    |     if axis == 1 
    |         for ii = coord(1):coord(end)
    |                 cubeout(ii,:,:) = cubei;
    |         end
    |     % draw normal to y-axis, i.e. in x-z plane
    |     elseif axis == 2
    |             for ii = coord(1):coord(end)
    |                 cubeout(:,ii,:) = cubei;
    |             end
    |     % draw normal to z-axis, i.e. in x-y plane
    |     elseif axis == 3;
    |             for ii = coord(1):coord(end)
    |                 cubeout(:,:,ii) = cubei;
    |             end
    |     end
  function cubeout = drawHeartBeat(axis,coord):
    | function cubeout = drawHeartBeat(axis,coord)
    |     cubeout = false(7,7,7);
    |     cubei = [0 0 0 0 0 0 0
    |               0 1 1 0 1 1 0;
    |               1 1 1 1 1 1 1;
    |               1 1 1 1 1 1 1;
    |               0 1 1 1 1 1 0;
    |               0 0 1 1 1 0 0;
    |               0 0 0 1 0 0 0];
    |      cubei = rot90(cubei,3);
    |      cubeib = [0 0 0 0 0 0 0;
    |                 0 0 0 0 0 0 0;
    |                 0 1 1 0 1 1 0;
    |                 0 1 1 1 1 1 0;
    |                 0 0 1 1 1 0 0;
    |                 0 0 0 0 0 0 0;
    |                 0 0 0 0 0 0 0];
    |      cubeib = rot90(cubeib,3);       
    |     % draw normal to x axis, i.e. in y-z plane
    |     if axis == 1 
    |         cubeout(coord-1,:,:) = cubeib;
    |         cubeout(coord,:,:) = cubei;
    |         cubeout(coord+1,:,:) = cubeib;
    |     % draw normal to y-axis, i.e. in x-z plane
    |     elseif axis == 2
    |         cubeout(:,coord-1,:) = cubeib;
    |         cubeout(:,coord,:) = cubei;
    |         cubeout(:,coord+1,:) = cubeib;
    |     % draw normal to z-axis, i.e. in x-y plane
    |     elseif axis == 3;
    |         cubeout(:,:,coord-1) = cubeib;
    |         cubeout(:,:,coord) = cubei;
    |         cubeout(:,:,coord+1) = cubeib;
    |     end
  function explosion = drawExplosion:
    | function explosion = drawExplosion
    | explosion = false(7,7,7);
    | % explosioni = logical([1     1     1     0     1     1     1;
    | %      1     1     0     1     0     1     1;
    | %      0     1     0     1     1     0     0;
    | %      1     0     1     1     0     1     0;
    | %      1     1     1     1     0     0     0;
    | %      0     1     1     1     0     0     1;
    | %      0     0     1     0     0     0     1]);
    |  
    | explosion(:,:,1) = logical([1     1     1     0     1     1     1;
    |      1     1     0     1     0     1     1;
    |      0     1     0     1     1     0     0;
    |      1     0     1     1     0     1     0;
    |      1     1     1     1     0     0     0;
    |      0     1     1     1     0     0     1;
    |      0     0     1     0     0     0     1]);
    | explosion(:,:,2) = fliplr(explosion(:,:,1));
    | explosion(:,:,3) = explosion(:,:,2)';
    | explosion(:,:,4) = explosion(:,:,1)';
    | explosion(:,:,5) = fliplr(explosion(:,:,3));
    | explosion(:,:,6) = explosion(:,:,2)';
    | explosion(:,:,7) = fliplr(explosion(:,:,3));
  function cubeOut = fireworks(cubeIn,step,explosion):
    | function cubeOut = fireworks(cubeIn,step,explosion)
    | cubeOut   = cubeIn;
    | % rocket states
    | if(step == 1)
    |   cubeOut(:) = 0;
    | elseif(step == 2)
    |   cubeOut(4,4,1) = 1;
    | elseif(step == 3)
    |   cubeOut(4,4,1) = 0;
    |   cubeOut(4,4,2) = 1;
    | elseif(step == 4)
    |   cubeOut(4,4,2) = 0;
    |   cubeOut(4,4,3) = 1;
    | elseif(step == 5)
    |   cubeOut(4,4,3) = 0;
    |   cubeOut(4,4,4) = 1;
    | elseif(step == 6)
    |   cubeOut(4,4,4) = 0;
    |   cubeOut(4,4,5) = 1;
    | elseif(step == 7)
    |   cubeOut(4,4,5) = 0;
    |   cubeOut(4,4,6) = 1;
    | elseif(step == 8)
    |   cubeOut(4,4,6) = 0;
    |   cubeOut(4,4,7) = 1;
    | % explosion states
    | elseif(step == 9)
    | %   explosion = logical(round(rand(7,7,7)));
    | %   mask      = false(7,7,7);    
    | %   mask(3:5,4,4) = 1; 
    | %   mask(4,3:5,4) = 1;
    | %   mask(4,4,3:5) = 1;
    | %   cubeOut = logical(mask.*explosion);
    |   cubeOut = false(7,7,7);
    |   cubeOut(3:5,4,4) = explosion(3:5,4,4);
    |   cubeOut(4,3:5,4) = explosion(4,3:5,4);
    |   cubeOut(4,4,3:5) = explosion(4,4,3:5);
    | elseif(step == 10)
    | %   explosion = logical(round(rand(7,7,7)));
    | %   mask      = false(7,7,7);  
    | %   mask(3:5,3:5,3:5) = 1;
    | %   cubeOut = logical(mask.*explosion);
    |     cubeOut = false(7,7,7);
    |     cubeOut(3:5,3:5,3:5) = explosion(3:5,3:5,3:5);
    | elseif(step == 11)
    | %   explosion = logical(round(rand(7,7,7)));
    | %   mask      = false(7,7,7);
    | %   mask(3:5,3:5,3:5) = 1;
    | %   mask(2:6,4,4) = 1;
    | %   mask(4,2:6,4) = 1;
    | %   mask(4,4,2:6) = 1;
    | %   cubeOut = logical(mask.*explosion);
    |     cubeOut = false(7,7,7);
    |     cubeOut(2:6,4,4) = explosion(2:6,4,4);
    |     cubeOut(4,2:6,4) = explosion(4,2:6,4);
    |     cubeOut(4,4,2:6) = explosion(4,4,2:6);
    | elseif(step == 12)
    | %   explosion = logical(round(rand(7,7,7)));
    | %   mask      = false(7,7,7);  
    | %   mask(3:5,2:6,3:5) = 1;
    | %   mask(3:5,3:5,2:6) = 1;
    | %   mask(2:6,3:5,3:5) = 1;
    | %   cubeOut = logical(mask.*explosion);
    |     cubeOut = false(7,7,7);
    |     cubeOut(2:6,3:5,3:5) = 1;
    |     cubeOut(3:5,2:6,3:5) = 1;
    |     cubeOut(3:5,3:5,2:6) = 1;
    | elseif(step == 13)
    | %   explosion = logical(round(rand(7,7,7)));
    | %   mask      = false(7,7,7);    
    | %   mask(2:6,2:6,2:6) = 1;
    | %   mask(4,:,4) = 1;
    | %   mask(4,4,:) = 1;
    | %   mask(:,4,4) = 1;
    | %   cubeOut = logical(mask.*explosion);
    |     cubeOut = false(7,7,7);
    |     cubeOut(2:6,2:6,2:6) = 1;
    |     cubeOut(:,4,4) = 1;
    |     cubeOut(4,:,4) = 1;
    |     cubeOut(4,4,:) = 1;
    | elseif(step == 14)
    | %   explosion = logical(round(rand(7,7,7)));
    | %   mask      = false(7,7,7);  
    |   % peak of explosion
    | %   cubeOut = logical(mask.*explosion);
    |     cubeOut = explosion;
    | else                                   % let the particles fall for 7 steps
    | %   cubeOut = logical(round(rand(7,7,7)));
    |   cubeOut(:,:,22-step:7) = 0;
    | end
    | end

== stateflow chart test_7x7x7_timing/State Machine1 ==
  state Firecrackers
    state LongWait
    state EvolveAnimation
      entry:
      cube = fireworks(cube,rStep,exp);
      exit:
      rStep = mod(rStep,21)+1;
    state ShortWait
      % Explosion
    (default) -> LongWait : {cube  = false(7,7,7);
        | exp = logical(round(rand(7,7,7)));
        | rStep = 1;}
    EvolveAnimation -> ShortWait [order 2] : [rStep > 8 && rStep < 15]
    LongWait -> EvolveAnimation : [after(0.1,sec)]
    ShortWait -> EvolveAnimation : [after(0.10,sec)]
    EvolveAnimation -> LongWait [order 1] : [rStep < 9 || rStep >14]
  state debug
  (default) -> (junction 466)
  (junction 461) -> ?
  (junction 466) -> Firecrackers [order 1] : [mode==9]
  (junction 466) -> debug [order 2]
  Firecrackers -> (junction 461) : [mode~=9]
  data: cubeIn function_input; step function_input; cubeOut function_output; explosion function_input; mode input; ledxyz input; cube output size=[7 7 7]; yi local; xi local; ledx input; ledy input; ledz input; rStep local; j local; i local; exp local
  function cubeOut = fireworks(cubeIn,step,explosion):
    | function cubeOut = fireworks(cubeIn,step,explosion)
    | cubeOut   = cubeIn;
    | % rocket states
    | if(step == 1)
    |   cubeOut(:) = 0;
    | elseif(step == 2)
    |   cubeOut(4,4,1) = 1;
    | elseif(step == 3)
    |   cubeOut(4,4,1) = 0;
    |   cubeOut(4,4,2) = 1;
    | elseif(step == 4)
    |   cubeOut(4,4,2) = 0;
    |   cubeOut(4,4,3) = 1;
    | elseif(step == 5)
    |   cubeOut(4,4,3) = 0;
    |   cubeOut(4,4,4) = 1;
    | elseif(step == 6)
    |   cubeOut(4,4,4) = 0;
    |   cubeOut(4,4,5) = 1;
    | elseif(step == 7)
    |   cubeOut(4,4,5) = 0;
    |   cubeOut(4,4,6) = 1;
    | elseif(step == 8)
    |   cubeOut(4,4,6) = 0;
    |   cubeOut(4,4,7) = 1;
    | % % explosion states
    | % elseif(step == 9)
    | % %   explosion = logical(round(rand(7,7,7)));
    | % %   mask      = false(7,7,7);    
    | % %   mask(3:5,4,4) = 1; 
    | % %   mask(4,3:5,4) = 1;
    | % %   mask(4,4,3:5) = 1;
    | % %   cubeOut = logical(mask.*explosion);
    | %   cubeOut = false(7,7,7);
    | %   cubeOut(3:5,4,4) = explosion(3:5,4,4);
    | %   cubeOut(4,3:5,4) = explosion(4,3:5,4);
    | %   cubeOut(4,4,3:5) = explosion(4,4,3:5);
    | % elseif(step == 10)
    | % %   explosion = logical(round(rand(7,7,7)));
    | % %   mask      = false(7,7,7);  
    | % %   mask(3:5,3:5,3:5) = 1;
    | % %   cubeOut = logical(mask.*explosion);
    | %     cubeOut(3:5,3:5,3:5) = explosion(3:5,3:5,3:5);
    | % elseif(step == 11)
    | % %   explosion = logical(round(rand(7,7,7)));
    | %   mask      = false(7,7,7);
    | %   mask(3:5,3:5,3:5) = 1;
    | %   mask(2:6,4,4) = 1;
    | %   mask(4,2:6,4) = 1;
    | %   mask(4,4,2:6) = 1;
    | %   cubeOut = logical(mask.*explosion);
    | % elseif(step == 12)
    | % %   explosion = logical(round(rand(7,7,7)));
    | %   mask      = false(7,7,7);  
    | %   mask(3:5,2:6,3:5) = 1;
    | %   mask(3:5,3:5,2:6) = 1;
    | %   mask(2:6,3:5,3:5) = 1;
    | %   cubeOut = logical(mask.*explosion);
    | % elseif(step == 13)
    | % %   explosion = logical(round(rand(7,7,7)));
    | %   mask      = false(7,7,7);    
    | %   mask(2:6,2:6,2:6) = 1;
    | %   mask(4,:,4) = 1;
    | %   mask(4,4,:) = 1;
    | %   mask(:,4,4) = 1;
    | %   cubeOut = logical(mask.*explosion);
    | % elseif(step == 14)
    | % %   explosion = logical(round(rand(7,7,7)));
    | %   mask      = false(7,7,7);  
    | %   % peak of explosion
    | %   cubeOut = logical(mask.*explosion);  
    | % else                                   % let the particles fall for 7 steps
    | % %   cubeOut = logical(round(rand(7,7,7)));
    | %   cubeOut(:,:,22-step:7) = 0;
    | end
    | end

== stateflow chart test_7x7x7_timing/CubeMode Test ==
  state TestMode
    entry:
    mode = 8;
  state TurnOff
    entry: mode = 1;
  (default) -> TestMode
  TestMode -> TurnOff : after(60,sec)
  data: mode output
